simulink model "Stateflow_rover"  (R2024a)
settings: Solver=FixedStepDiscrete  StartTime=0.0  StopTime=10.0  FixedStep=0.001  RelTol=1e-3  EnableMultiTasking=on
settings Model: Creator=guido  LastModifiedBy=guido
settings SolverCC: AlgebraicLoopSolver=TrustRegion  AutoInsertRateTranBlk=on
settings DataIOCC: LimitDataPoints=on
settings OptimizationCC: DefaultParameterBehavior=Inlined  UseDivisionForNetSlopeComputation=on  GainParamInheritBuiltInType=on  UseFloatMulNetSlope=on  InlineInvariantSignals=on  PassReuseOutputArgsAs=Individual arguments  ZeroExternalMemoryAtStartup=off  ZeroInternalMemoryAtStartup=off  NoFixptDivByZeroProtection=on  EfficientFloat2IntCast=on  LifeSpan=1  OptimizeBlockOrder=speed  DifferentSizesBufferReuse=on  EfficientTunableParamExpr=on
settings DebuggingCC: ParameterTunabilityLossMsg=error  UnconnectedInputMsg=warning  UnconnectedOutputMsg=warning  UnconnectedLineMsg=warning  AllowSymbolicDim=off  SFUnexpectedBacktrackingDiag=warning  SFNoUnconditionalDefaultTransitionDiag=warning  SFExecutionAtInitializationDiag=none  ArithmeticOperatorsInVariantConditions=warning
settings HardwareCC: ProdLongLongMode=on
settings ModelReferenceCC: EnableRefExpFcnMdlSchedulingChecks=on
settings SFSimCC: SimUseLocalCustomCode=off  MATLABDynamicMemAlloc=off  CustomCodeUndefinedFunction=UseInterfaceOnly
settings RTWCC: Description=Embedded Coder  SystemTargetFile=ert.tlc  TemplateMakefile=ert_default_tmf  RTWUseLocalCustomCode=off  GPUComputeCapability=3.5  DLArmComputeVersion=19.05
settings CodeAppCC: ForceParamTrailComments=on  IgnoreCustomStorageClasses=off  OperatorAnnotations=on  SimulinkDataObjDesc=on  SFDataObjDesc=on  CustomSymbolStrGlobalVar=rt$N$M  CustomSymbolStrType=$N$M  CustomSymbolStrFcn=$N$M$F  CustomSymbolStrMacro=$N$M  InsertBlockDesc=on
settings ERTTargetCC: GenerateSampleERTMain=on  IncludeMdlTerminateFcn=off  CombineSignalStateStructs=on  SupportAbsoluteTime=off  SupportNonFinite=off  SupportComplex=off  SupportNonInlinedSFcns=on  InlinedParameterPlacement=NonHierarchical  ERTCustomFileTemplate=example_file_process.tlc  ERTFilePackagingFormat=CompactWithDataFile
settings ConfigComp: CovMetricSettings=dw  CovSaveCumulativeToWorkspaceVar=on  CovSaveSingleToWorkspaceVar=on  CovExternalEMLEnable=off  CovSFcnEnable=off

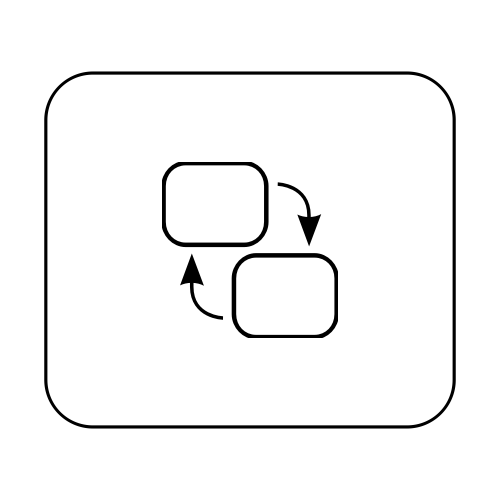
[thumbnail: Simulink's stored preview of the top-level diagram]
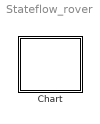
== system Stateflow_rover ==
  Chart : Stateflow chart  TreatAsAtomicUnit=on

== stateflow chart Stateflow_rover/Chart ==
  state ROVER
    state BOARD1 [parallel]
      settings: executionOrder=1
      state READ_TASK_B1
        state READ_OK
          (default) -> (junction 184)
          (junction 184) -> (junction 185) [order 1] : [Temp_B1 >=90 | Temp_B1 == 0]{countTempB1 = countTempB1 +1}
          (junction 184) -> (junction 185) [order 2] : {countTempB1 = 0}
        state START
          en: Enc1 = 0;
          en: Enc2 = 0;
          en: Enc3 = 0;
          en: Enc4 = 0;
          en: Temp_B1 = 0;
        (default) -> ROVER.BOARD1.READ_TASK_B1.START
        ROVER.BOARD1.READ_TASK_B1.START -> ROVER.BOARD1.READ_TASK_B1.READ_OK : {readEncs(); ...
            | TemperatureSensor_ReadB1()}
      state COMMUNICATION_TASK_B1
        state DECISION
        state SEND_DATA
        state START
          en: B2State_inB1 = 0;
          en:final_decisionB1 = 3;
          en: B1_decision = 4;
          en: Board_state = 3;
        state TIMEOUT
          en: Board_state = 1;
        state WAIT_B2
        state RECEIVE_FINAL_DECISION
        state CONTROL_DECISION
        ROVER.BOARD1.COMMUNICATION_TASK_B1.DECISION -> ROVER.BOARD1.COMMUNICATION_TASK_B1.SEND_DATA [order 1] : [B1State == 1 & B2State_inB1 == 0]
            | {Board_state = 0; B1_decision = 0}
        (default) -> ROVER.BOARD1.COMMUNICATION_TASK_B1.START
        ROVER.BOARD1.COMMUNICATION_TASK_B1.DECISION -> ROVER.BOARD1.COMMUNICATION_TASK_B1.SEND_DATA [order 2] : [B1State == 1 & B2State_inB1 == 1]
            | {Board_state = 1; B1_decision = 1}
        ROVER.BOARD1.COMMUNICATION_TASK_B1.DECISION -> ROVER.BOARD1.COMMUNICATION_TASK_B1.SEND_DATA [order 3] : [B2State_inB1 == 1]
            | {B1_decision = 2}
        ROVER.BOARD1.COMMUNICATION_TASK_B1.START -> ROVER.BOARD1.COMMUNICATION_TASK_B1.DECISION [order 1] : [B2_pin == 1]
            | {B1_pin = 1;
            | receiveB2();
            | B1_pin = 0
            | computeB1GlobalState()}
        ROVER.BOARD1.COMMUNICATION_TASK_B1.DECISION -> ROVER.BOARD1.COMMUNICATION_TASK_B1.SEND_DATA [order 4] : {B1_decision = 3}
        ROVER.BOARD1.COMMUNICATION_TASK_B1.SEND_DATA -> WAIT_B2 : {B1_pin = 1}
        ROVER.BOARD1.COMMUNICATION_TASK_B1.START -> ROVER.BOARD1.COMMUNICATION_TASK_B1.TIMEOUT [order 2] : [after(78, msec)]
        ROVER.BOARD1.COMMUNICATION_TASK_B1.TIMEOUT -> ROVER.BOARD1.COMMUNICATION_TASK_B1.START
        WAIT_B2 -> ROVER.BOARD1.COMMUNICATION_TASK_B1.TIMEOUT [order 2] : [after(10, msec)]
        RECEIVE_FINAL_DECISION -> ROVER.BOARD1.COMMUNICATION_TASK_B1.TIMEOUT [order 2] : [after(10,msec)]
        WAIT_B2 -> RECEIVE_FINAL_DECISION [order 1] : [B2_pin == 1]
            | {transmitB1();
            | B1_pin = 0;}
        RECEIVE_FINAL_DECISION -> ROVER.BOARD1.COMMUNICATION_TASK_B1.CONTROL_DECISION [order 1] : [B2_pin == 1]{B1_pin = 1;
            | receiveB2();
            | B1_pin = 0}
      state EMERGENCY_ACTUATION_TASK_B1
        state START
        state ACTUATION
        state END_EM
        (default) -> ROVER.BOARD1.EMERGENCY_ACTUATION_TASK_B1.START
        ROVER.BOARD1.EMERGENCY_ACTUATION_TASK_B1.START -> ROVER.BOARD1.EMERGENCY_ACTUATION_TASK_B1.ACTUATION [order 1] : [Board_state == 0]
        ROVER.BOARD1.EMERGENCY_ACTUATION_TASK_B1.START -> ROVER.BOARD1.EMERGENCY_ACTUATION_TASK_B1.END_EM [order 2]
        ROVER.BOARD1.EMERGENCY_ACTUATION_TASK_B1.ACTUATION -> ROVER.BOARD1.EMERGENCY_ACTUATION_TASK_B1.END_EM : {emergencyActuation()}
      state ACTUATION_TASK_B1
        state ACTUATION
        state START1
        state END_ACT
        (default) -> ROVER.BOARD1.ACTUATION_TASK_B1.START1
        ROVER.BOARD1.ACTUATION_TASK_B1.START1 -> ROVER.BOARD1.ACTUATION_TASK_B1.ACTUATION [order 1] : [Board_state == 1]
        ROVER.BOARD1.ACTUATION_TASK_B1.ACTUATION -> ROVER.BOARD1.ACTUATION_TASK_B1.END_ACT : {Actuation();}
        ROVER.BOARD1.ACTUATION_TASK_B1.START1 -> ROVER.BOARD1.ACTUATION_TASK_B1.END_ACT [order 2]
      (default) -> READ_TASK_B1
      ROVER.BOARD1.READ_TASK_B1.READ_OK -> COMMUNICATION_TASK_B1 [order 2] : {B1State = 1;
          | createB1PartialState()}
      ROVER.BOARD1.READ_TASK_B1.READ_OK -> COMMUNICATION_TASK_B1 [order 1] : [Enc1 < 0 | Enc2 < 0 | Enc3 < 0 | Enc4 < 0 | countTempB1 > 200]
          | {B1State = 0;
          | createB1PartialState()}
      ROVER.BOARD1.EMERGENCY_ACTUATION_TASK_B1.END_EM -> READ_TASK_B1
      ROVER.BOARD1.COMMUNICATION_TASK_B1.CONTROL_DECISION -> ACTUATION_TASK_B1 [order 2] : {Board_state = 3}
      ROVER.BOARD1.COMMUNICATION_TASK_B1.CONTROL_DECISION -> ACTUATION_TASK_B1 [order 1] : [final_decisionB1 == 1]
      ROVER.BOARD1.ACTUATION_TASK_B1.END_ACT -> EMERGENCY_ACTUATION_TASK_B1
    state BOARD2 [parallel]
      settings: executionOrder=2
      state READ_TASK_B2
        state READ_OK
          (default) -> (junction 202)
          (junction 202) -> (junction 200) [order 1] : [Temp_B2 >= 90 | Temp_B2 == 0]{countTempB2 = countTempB2 +1}
          (junction 202) -> (junction 200) [order 2] : {countTempB2 = 0}
        state START
          en: sonar1 = 0;
          en: sonar2 = 0;
          en: sonar3 = 0;
          en: PSX_LF = 0;
          en: PSX_RS = 0;
          en: Red_Btn = 0;
          en: Black_Btn = 0;
          en: Temp_B2 = 0;
        (default) -> ROVER.BOARD2.READ_TASK_B2.START
        ROVER.BOARD2.READ_TASK_B2.START -> ROVER.BOARD2.READ_TASK_B2.READ_OK : {readSonar();
            | TemperatureSensor_ReadB2();
            | readController();
            | readAcc();}
      state COMMUNICATION_TASK_B2
        state DECISION
        state START
          en: StatusBoardB2 = 0;
          en: B1State_inB2 = 0;
          en: B2Decision = 4;
          en: final_decisionB2 = 3;
        state SEND_DATA
        state RECEIVE_DATA
        state TIMEOUT
          en :StatusBoardB2 = 0;
        state COMPUTE_FINAL_DECISION
        state END_COMM
        state CONTROL2
        state SEND_FINAL_DECISION
        state SEND_FINAL_DECISION1
        state CONTROL_DECISION
        (default) -> ROVER.BOARD2.COMMUNICATION_TASK_B2.START
        ROVER.BOARD2.COMMUNICATION_TASK_B2.SEND_DATA -> RECEIVE_DATA [order 1] : [B1_pin == 1]
            | {transmitB2();
            | B2_pin = 0}
        RECEIVE_DATA -> ROVER.BOARD2.COMMUNICATION_TASK_B2.DECISION [order 1] : [B1_pin == 1]
            | {B2_pin = 1;
            | receiveB1();
            | B2_pin = 0;
            | computeB2GlobalState()}
        ROVER.BOARD2.COMMUNICATION_TASK_B2.DECISION -> COMPUTE_FINAL_DECISION [order 4] : {B2_decision = 3;
            | StatusBoardB2 = 0}
        RECEIVE_DATA -> ROVER.BOARD2.COMMUNICATION_TASK_B2.TIMEOUT [order 2] : [after(10,msec)]
        ROVER.BOARD2.COMMUNICATION_TASK_B2.DECISION -> COMPUTE_FINAL_DECISION [order 1] : [B1State_inB2 == 1 & B2State == 0]
            | {B2_decision = 0}
        ROVER.BOARD2.COMMUNICATION_TASK_B2.DECISION -> COMPUTE_FINAL_DECISION [order 2] : [B1State_inB2 == 1 & B2State == 1]
            | {B2_decision = 1}
        ROVER.BOARD2.COMMUNICATION_TASK_B2.DECISION -> COMPUTE_FINAL_DECISION [order 3] : [B2State == 1]
            | {B2_decision = 0;
            | StatusBoardB2 = 1}
        ROVER.BOARD2.COMMUNICATION_TASK_B2.START -> ROVER.BOARD2.COMMUNICATION_TASK_B2.SEND_DATA : {B2_pin = 1}
        ROVER.BOARD2.COMMUNICATION_TASK_B2.SEND_DATA -> ROVER.BOARD2.COMMUNICATION_TASK_B2.TIMEOUT [order 2] : [after(10,msec)]
        SEND_FINAL_DECISION1 -> ROVER.BOARD2.COMMUNICATION_TASK_B2.TIMEOUT [order 2] : [after(10,msec)]
        CONTROL2 -> END_COMM [order 2] : {StatusBoardB2 = 0}
        CONTROL2 -> END_COMM [order 1] : [B2State == 1]
            | {StatusBoardB2 = 1}
        COMPUTE_FINAL_DECISION -> SEND_FINAL_DECISION [order 1] : [B1_decision == B2_decision]
            | {final_decisionB2 = 1}
        COMPUTE_FINAL_DECISION -> SEND_FINAL_DECISION [order 2] : {final_decisionB2 = 0}
        ROVER.BOARD2.COMMUNICATION_TASK_B2.CONTROL_DECISION -> END_COMM [order 1] : [final_decisionB2 == 1]
        ROVER.BOARD2.COMMUNICATION_TASK_B2.CONTROL_DECISION -> CONTROL2 [order 2]
        SEND_FINAL_DECISION -> SEND_FINAL_DECISION1 : {B2_pin = 1}
        SEND_FINAL_DECISION1 -> ROVER.BOARD2.COMMUNICATION_TASK_B2.CONTROL_DECISION [order 1] : [B1_pin == 1]
            | {transmitDecision();
            | B2_pin = 0}
      state DEGRADATED_ACTUATION_TASK_B2
        state ACTUATION
        state START1
        state END_ACT
        ROVER.BOARD2.DEGRADATED_ACTUATION_TASK_B2.START1 -> ROVER.BOARD2.DEGRADATED_ACTUATION_TASK_B2.ACTUATION [order 1] : [StatusBoardB2 == 1]
        (default) -> ROVER.BOARD2.DEGRADATED_ACTUATION_TASK_B2.START1
        ROVER.BOARD2.DEGRADATED_ACTUATION_TASK_B2.ACTUATION -> ROVER.BOARD2.DEGRADATED_ACTUATION_TASK_B2.END_ACT : {DegActuation()}
        ROVER.BOARD2.DEGRADATED_ACTUATION_TASK_B2.START1 -> ROVER.BOARD2.DEGRADATED_ACTUATION_TASK_B2.END_ACT [order 2]
      state EMERGENCY_ACTUATION_TASK_B2
        state ACTUATION
        state START
        state END_EM
        (default) -> ROVER.BOARD2.EMERGENCY_ACTUATION_TASK_B2.START
        ROVER.BOARD2.EMERGENCY_ACTUATION_TASK_B2.START -> ROVER.BOARD2.EMERGENCY_ACTUATION_TASK_B2.ACTUATION [order 1] : [StatusBoardB2 == 1]
        ROVER.BOARD2.EMERGENCY_ACTUATION_TASK_B2.ACTUATION -> ROVER.BOARD2.EMERGENCY_ACTUATION_TASK_B2.END_EM : {emergencyActuation()}
        ROVER.BOARD2.EMERGENCY_ACTUATION_TASK_B2.START -> ROVER.BOARD2.EMERGENCY_ACTUATION_TASK_B2.END_EM [order 2]
      (default) -> READ_TASK_B2
      ROVER.BOARD2.READ_TASK_B2.READ_OK -> COMMUNICATION_TASK_B2 [order 2] : {B2State = 1;
          | createB2PartialState()}
      ROVER.BOARD2.READ_TASK_B2.READ_OK -> COMMUNICATION_TASK_B2 [order 1] : [sonar1 < 0 | sonar2 < 0 | sonar3 < 0 | PSX_LF <= 0 | PSX_RS <= 0 | countTempB2 > 200]
          | {B2State = 0;
          | createB2PartialState()}
      ROVER.BOARD2.EMERGENCY_ACTUATION_TASK_B2.END_EM -> READ_TASK_B2
      END_COMM -> DEGRADATED_ACTUATION_TASK_B2
      ROVER.BOARD2.DEGRADATED_ACTUATION_TASK_B2.END_ACT -> EMERGENCY_ACTUATION_TASK_B2
  (default) -> ROVER
  data: Black_Btn local; B1State local; B2State local; Enc1 local; Enc2 local; Enc3 local; Enc4 local; PSX_LF local; PSX_RS local; Red_Btn local; Temp_B1 local; Temp_B2 local; countTempB1 local; countTempB2 local; sonar1 local; sonar2 local; sonar3 local; B1State_inB2 local; B2State_inB1 local; countAckB1 local; countAckB2 local; StartActB1 local; StatusBoardB3 local; StartEmergencyB1 local; StatusBoardB2 local; CommReadyB2 local; CommReadyB1 local; B2_CTS local; B1_CTS local; B2Decision local; B1_decision local; B1_pin local; B2_decision local; B2_pin local; Board_state local; final_decisionB1 local; final_decisionB2 local
  function Actuation:
    | function Actuation
  function TemperatureSensor_ReadB2:
    | function TemperatureSensor_ReadB2
  function transmitDecision:
    | function transmitDecision
  function createB1PartialState:
    | function createB1PartialState
  function createB2PartialState:
    | function createB2PartialState
  function emergencyActuation:
    | function emergencyActuation
  function DegActuation:
    | function DegActuation
  function TemperatureSensor_ReadB1:
    | function TemperatureSensor_ReadB1
  function transmitB1:
    | function transmitB1
  function transmitB2:
    | function transmitB2
  function readController:
    | function readController
  function readAcc:
    | function readAcc
  function readEncs:
    | function readEncs
  function readSonar:
    | function readSonar
  function computeB1GlobalState:
    | function computeB1GlobalState
  function computeB2GlobalState:
    | function computeB2GlobalState
  function receiveB1:
    | function receiveB1
  function receiveB2:
    | function receiveB2
